simulink model "usv_model"  (R2015b)
settings: Solver=ode45  StartTime=0.0  StopTime=100000.0  RelTol=1e-3
model workspace (MAT data in the model file):
  B = 3.17
  Cb = 0.251
  Izz = 1
  L = 9.8
  d = 0.71
  m = 5540
undefined symbols (not defined in the file or in its folder): magnitude
libraries: simulink x2
settings Model: Creator=Administrator  LastModifiedBy=Administrator

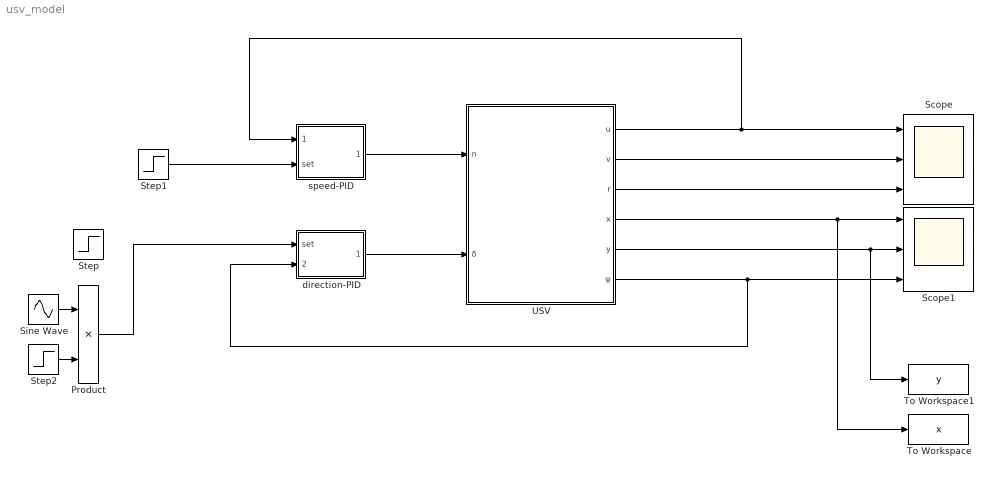
== system usv_model ==
  Product : Product
  Scope : Scope  NumInputPorts=3
  Scope1 : Scope  NumInputPorts=3
  Sine Wave : Sin  Amplitude=90  Frequency=1/5000  SampleTime=0
  Step : Step  Time=30000  After=50  SampleTime=0
  Step1 : Step  Time=0  After=0.1  SampleTime=0
  Step2 : Step  Time=60000  SampleTime=0
  To Workspace : ToWorkspace  VariableName=x  SampleTime=-1
  To Workspace1 : ToWorkspace  VariableName=y  SampleTime=-1
  USV : Subsystem
  direction-PID : Subsystem
  speed-PID : Subsystem
  wires:
  USV/5(y) -> To Workspace1/1, Scope1/2
  USV/4(x) -> To Workspace/1, Scope1/1
  USV/1(u) -> speed-PID/1(feedback), Scope/1
  USV/2(v) -> Scope/2
  USV/3(r) -> Scope/3
  USV/6(ψ) -> direction-PID/2(feedback), Scope1/3
  Sine Wave/1 -> Product/1
  Step2/1 -> Product/2
  Step1/1 -> speed-PID/2(set)
  speed-PID/1(output) -> USV/1(n)
  Product/1 -> direction-PID/1(set)
  direction-PID/1(output) -> USV/2(δ)

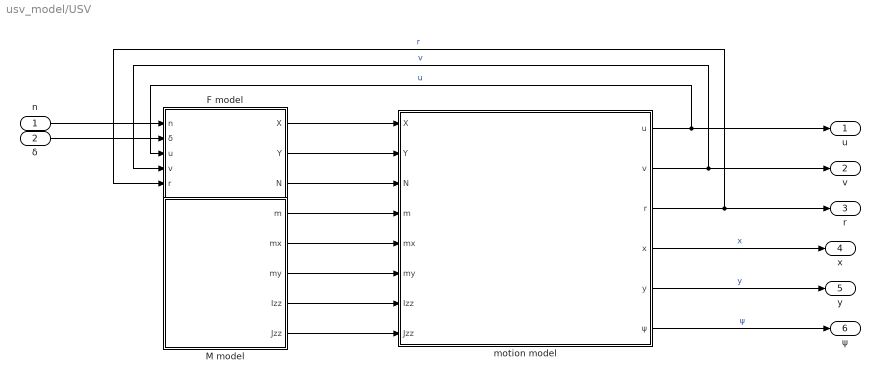
== system usv_model/USV ==
  n : Inport
  δ : Inport  Port=2
  F model : Subsystem
  M model : Subsystem
  motion model : Subsystem
  u : Outport
  v : Outport  Port=2
  r : Outport  Port=3
  x : Outport  Port=4
  y : Outport  Port=5
  ψ : Outport  Port=6
  wires:
  M model/5(Jzz) -> motion model/8(Jzz)
  M model/3(my) -> motion model/6(my)
  M model/1(m) -> motion model/4(m)
  F model/2(Y) -> motion model/2(Y)
  n/1 -> F model/1(n)
  δ/1 -> F model/2(δ)
  F model/1(X) -> motion model/1(X)
  motion model/1(u) -> u/1, F model/3(u)  "u"
  motion model/3(r) -> r/1, F model/5(r)  "r"
  motion model/2(v) -> v/1, F model/4(v)  "v"
  motion model/6(ψ) -> ψ/1  "ψ"
  F model/3(N) -> motion model/3(N)
  M model/2(mx) -> motion model/5(mx)
  M model/4(Izz) -> motion model/7(Izz)
  motion model/4(x) -> x/1  "x"
  motion model/5(y) -> y/1  "y"

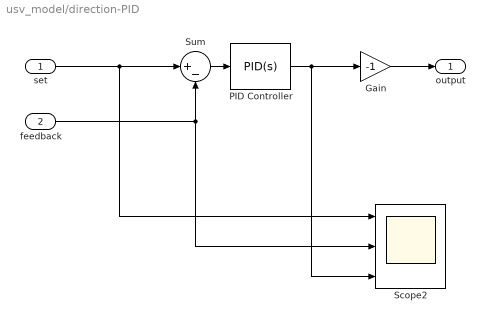
== system usv_model/direction-PID ==
  set : Inport
  feedback : Inport  Port=2
  Gain : Gain  Gain=-1
  PID Controller : simulink/Continuous/PID Controller  Controller=PID  TimeDomain=Continuous-time  SampleTime=-1  IntegratorMethod=Forward Euler  FilterMethod=Forward Euler  Form=Parallel  UseFilter=on  ControllerParametersSource=internal  P=1.2  I=0  D=0  N=5.45397025421619  InitialConditionSource=internal  InitialConditionForIntegrator=0  InitialConditionForFilter=0  ExternalReset=none  LimitOutput=on  UpperSaturationLimit=50  LowerSaturationLimit=-50  LinearizeAsGain=on  AntiWindupMode=none  Kb=1  TrackingMode=off  Kt=1  PParamMin=[]  PParamMax=[]  IParamMin=[]  IParamMax=[]  DParamMin=[]  DParamMax=[]  NParamMin=[]  NParamMax=[]  KbParamMin=[]  KbParamMax=[]  KtParamMin=[]  KtParamMax=[]  POutMin=[]  POutMax=[]  IOutMin=[]  IOutMax=[]  DOutMin=[]  DOutMax=[]  NOutMin=[]  NOutMax=[]  KbOutMin=[]  KbOutMax=[]  KtOutMin=[]  KtOutMax=[]  IntegratorOutMin=[]  IntegratorOutMax=[]  FilterOutMin=[]  FilterOutMax=[]  SumOutMin=[]  SumOutMax=[]  SumI1OutMin=[]  SumI1OutMax=[]  SumI2OutMin=[]  SumI2OutMax=[]  SumI3OutMin=[]  SumI3OutMax=[]  SumDOutMin=[]  SumDOutMax=[]  SaturationOutMin=[]  SaturationOutMax=[]  IntegratorContinuousStateAttributes=''  IntegratorStateMustResolveToSignalObject=off  IntegratorRTWStateStorageClass=Auto  FilterContinuousStateAttributes=''  FilterStateMustResolveToSignalObject=off  FilterRTWStateStorageClass=Auto  DifferentiatorICPrevScaledInput=0  DifferentiatorOutMin=[]  DifferentiatorOutMax=[]
  Scope2 : Scope  NumInputPorts=3
  Sum : Sum  Inputs=|+-
  output : Outport
  wires:
  PID Controller/1 -> Gain/1, Scope2/3
  Sum/1 -> PID Controller/1
  set/1 -> Scope2/1, Sum/1
  feedback/1 -> Scope2/2, Sum/2
  Gain/1 -> output/1

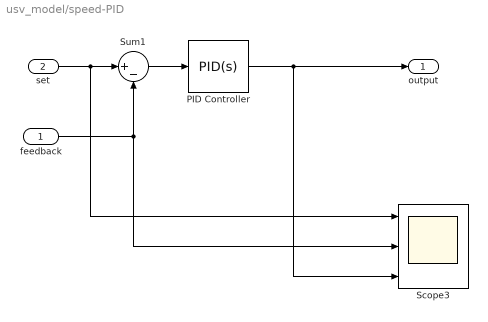
== system usv_model/speed-PID ==
  feedback : Inport
  set : Inport  Port=2
  PID Controller : simulink/Continuous/PID Controller  Controller=PID  TimeDomain=Continuous-time  SampleTime=-1  IntegratorMethod=Forward Euler  FilterMethod=Forward Euler  Form=Parallel  UseFilter=on  ControllerParametersSource=internal  P=3000  I=2  D=0  N=5.45397025421619  InitialConditionSource=internal  InitialConditionForIntegrator=0  InitialConditionForFilter=0  ExternalReset=none  LimitOutput=on  UpperSaturationLimit=2000  LowerSaturationLimit=0  LinearizeAsGain=on  AntiWindupMode=none  Kb=1  TrackingMode=off  Kt=1  PParamMin=[]  PParamMax=[]  IParamMin=[]  IParamMax=[]  DParamMin=[]  DParamMax=[]  NParamMin=[]  NParamMax=[]  KbParamMin=[]  KbParamMax=[]  KtParamMin=[]  KtParamMax=[]  POutMin=[]  POutMax=[]  IOutMin=[]  IOutMax=[]  DOutMin=[]  DOutMax=[]  NOutMin=[]  NOutMax=[]  KbOutMin=[]  KbOutMax=[]  KtOutMin=[]  KtOutMax=[]  IntegratorOutMin=[]  IntegratorOutMax=[]  FilterOutMin=[]  FilterOutMax=[]  SumOutMin=[]  SumOutMax=[]  SumI1OutMin=[]  SumI1OutMax=[]  SumI2OutMin=[]  SumI2OutMax=[]  SumI3OutMin=[]  SumI3OutMax=[]  SumDOutMin=[]  SumDOutMax=[]  SaturationOutMin=[]  SaturationOutMax=[]  IntegratorContinuousStateAttributes=''  IntegratorStateMustResolveToSignalObject=off  IntegratorRTWStateStorageClass=Auto  FilterContinuousStateAttributes=''  FilterStateMustResolveToSignalObject=off  FilterRTWStateStorageClass=Auto  DifferentiatorICPrevScaledInput=0  DifferentiatorOutMin=[]  DifferentiatorOutMax=[]
  Scope3 : Scope  NumInputPorts=3
  Sum1 : Sum  Inputs=|+-
  output : Outport
  wires:
  set/1 -> Sum1/1, Scope3/1
  PID Controller/1 -> output/1, Scope3/3
  Sum1/1 -> PID Controller/1
  feedback/1 -> Sum1/2, Scope3/2

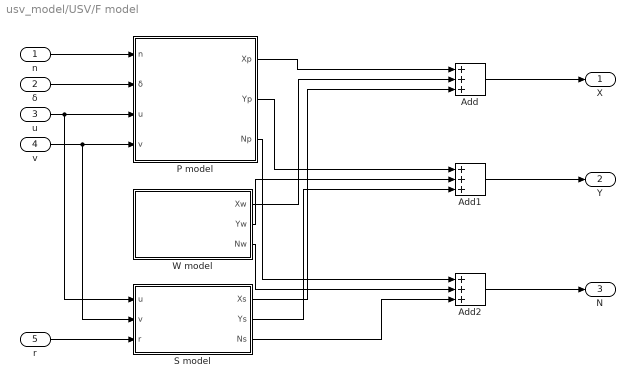
== system usv_model/USV/F model ==
  n : Inport
  δ : Inport  Port=2
  u : Inport  Port=3
  v : Inport  Port=4
  r : Inport  Port=5
  Add : Sum  Inputs=3
  Add1 : Sum  Inputs=3
  Add2 : Sum  Inputs=3
  P model : Subsystem
  S model : Subsystem
  W model : Subsystem
  X : Outport
  Y : Outport  Port=2
  N : Outport  Port=3
  wires:
  n/1 -> P model/1(n)
  δ/1 -> P model/2(δ)
  P model/1(Xp) -> Add/1
  W model/1(Xw) -> Add/2
  S model/1(Xs) -> Add/3
  P model/2(Yp) -> Add1/1
  W model/2(Yw) -> Add1/2
  S model/2(Ys) -> Add1/3
  P model/3(Np) -> Add2/1
  W model/3(Nw) -> Add2/2
  S model/3(Ns) -> Add2/3
  Add/1 -> X/1
  Add1/1 -> Y/1
  Add2/1 -> N/1
  u/1 -> S model/1(u), P model/3(u)
  v/1 -> S model/2(v), P model/4(v)
  r/1 -> S model/3(r)

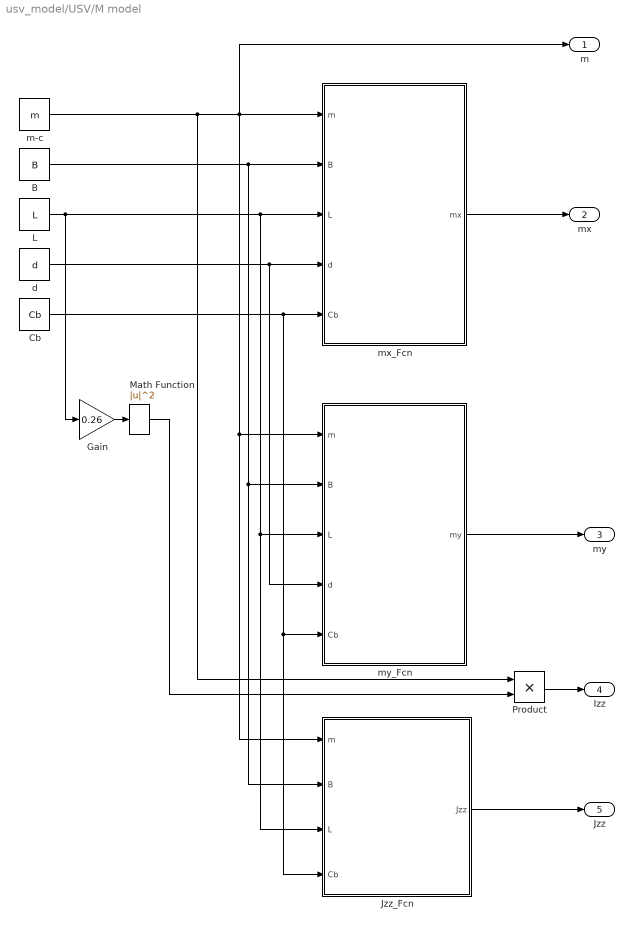
== system usv_model/USV/M model ==
  B : Constant  Value=B
  Cb : Constant  Value=Cb
  Gain : Gain  Gain=0.26
  Jzz_Fcn : MATLAB Function  TreatAsAtomicUnit=on
  L : Constant  Value=L
  Math Function : Math  Operator=magnitude^2  SaturateOnIntegerOverflow=on
  Product : Product
  d : Constant  Value=d
  m-c : Constant  Value=m
  mx_Fcn : MATLAB Function  TreatAsAtomicUnit=on
  my_Fcn : MATLAB Function  TreatAsAtomicUnit=on
  m : Outport
  mx : Outport  Port=2
  my : Outport  Port=3
  Izz : Outport  Port=4
  Jzz : Outport  Port=5
  wires:
  mx_Fcn/1(mx) -> mx/1
  d/1 -> my_Fcn/4(d), mx_Fcn/4(d)
  B/1 -> Jzz_Fcn/2(B), my_Fcn/2(B), mx_Fcn/2(B)
  my_Fcn/1(my) -> my/1
  Jzz_Fcn/1(Jzz) -> Jzz/1
  m-c/1 -> Product/1, m/1, Jzz_Fcn/1(m), my_Fcn/1(m), mx_Fcn/1(m)
  L/1 -> Gain/1, Jzz_Fcn/3(L), my_Fcn/3(L), mx_Fcn/3(L)
  Cb/1 -> Jzz_Fcn/4(Cb), my_Fcn/5(Cb), mx_Fcn/5(Cb)
  Gain/1 -> Math Function/1
  Product/1 -> Izz/1
  Math Function/1 -> Product/2

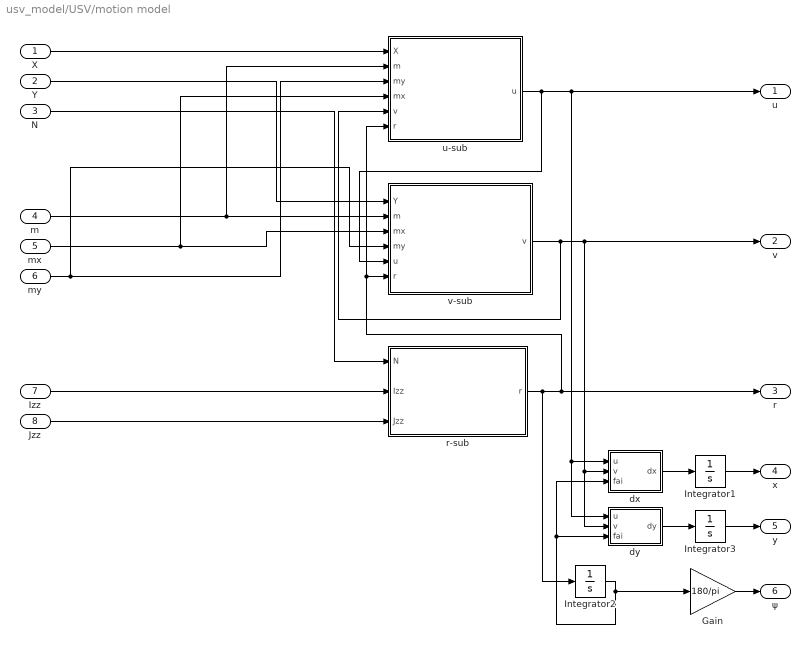
== system usv_model/USV/motion model ==
  X : Inport
  Y : Inport  Port=2
  N : Inport  Port=3
  m : Inport  Port=4
  mx : Inport  Port=5
  my : Inport  Port=6
  Izz : Inport  Port=7
  Jzz : Inport  Port=8
  Gain : Gain  Gain=180/pi
  Integrator1 : Integrator
  Integrator2 : Integrator
  Integrator3 : Integrator
  dx : MATLAB Function  TreatAsAtomicUnit=on
  dy : MATLAB Function  TreatAsAtomicUnit=on
  r-sub : Subsystem
  u-sub : Subsystem
  v-sub : Subsystem
  u : Outport
  v : Outport  Port=2
  r : Outport  Port=3
  x : Outport  Port=4
  y : Outport  Port=5
  ψ : Outport  Port=6
  wires:
  m/1 -> v-sub/2(m), u-sub/2(m)
  Y/1 -> v-sub/1(Y)
  r-sub/1(r) -> r/1, u-sub/6(r), v-sub/6(r), Integrator2/1
  Izz/1 -> r-sub/2(Izz)
  N/1 -> r-sub/1(N)
  Jzz/1 -> r-sub/3(Jzz)
  X/1 -> u-sub/1(X)
  my/1 -> u-sub/3(my), v-sub/4(my)
  mx/1 -> u-sub/4(mx), v-sub/3(mx)
  v-sub/1(v) -> dy/2(v), dx/2(v), v/1, u-sub/5(v)
  u-sub/1(u) -> u/1, dy/1(u), dx/1(u), v-sub/5(u)
  dy/1(dy) -> Integrator3/1
  dx/1(dx) -> Integrator1/1
  Integrator3/1 -> y/1
  Integrator1/1 -> x/1
  Gain/1 -> ψ/1
  Integrator2/1 -> Gain/1, dy/3(fai), dx/3(fai)

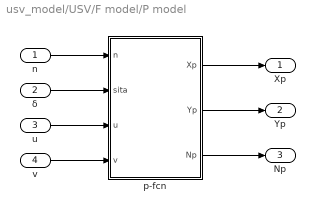
== system usv_model/USV/F model/P model ==
  n : Inport
  δ : Inport  Port=2
  u : Inport  Port=3
  v : Inport  Port=4
  p-fcn : MATLAB Function  TreatAsAtomicUnit=on
  Xp : Outport
  Yp : Outport  Port=2
  Np : Outport  Port=3
  wires:
  p-fcn/3(Np) -> Np/1
  p-fcn/2(Yp) -> Yp/1
  p-fcn/1(Xp) -> Xp/1
  n/1 -> p-fcn/1(n)
  δ/1 -> p-fcn/2(sita)
  u/1 -> p-fcn/3(u)
  v/1 -> p-fcn/4(v)

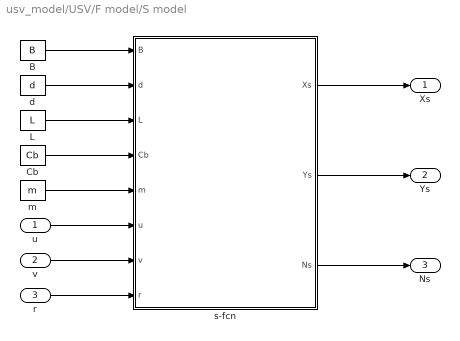
== system usv_model/USV/F model/S model ==
  u : Inport
  v : Inport  Port=2
  r : Inport  Port=3
  B : Constant  Value=B
  Cb : Constant  Value=Cb
  L : Constant  Value=L
  d : Constant  Value=d
  m : Constant  Value=m
  s-fcn : MATLAB Function  TreatAsAtomicUnit=on
  Xs : Outport
  Ys : Outport  Port=2
  Ns : Outport  Port=3
  wires:
  s-fcn/1(Xs) -> Xs/1
  s-fcn/2(Ys) -> Ys/1
  s-fcn/3(Ns) -> Ns/1
  B/1 -> s-fcn/1(B)
  d/1 -> s-fcn/2(d)
  L/1 -> s-fcn/3(L)
  u/1 -> s-fcn/6(u)
  v/1 -> s-fcn/7(v)
  r/1 -> s-fcn/8(r)
  Cb/1 -> s-fcn/4(Cb)
  m/1 -> s-fcn/5(m)

== system usv_model/USV/F model/W model ==
  n : Constant  Value=0
  n1 : Constant  Value=0
  n2 : Constant  Value=0
  Xw : Outport
  Yw : Outport  Port=2
  Nw : Outport  Port=3
  wires:
  n/1 -> Xw/1
  n2/1 -> Yw/1
  n1/1 -> Nw/1

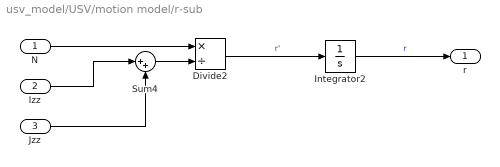
== system usv_model/USV/motion model/r-sub ==
  N : Inport
  Izz : Inport  Port=2
  Jzz : Inport  Port=3
  Divide2 : Product  Inputs=*/
  Integrator2 : Integrator
  Sum4 : Sum  Inputs=|++
  r : Outport
  wires:
  Sum4/1 -> Divide2/2
  Divide2/1 -> Integrator2/1  "r'"
  Integrator2/1 -> r/1  "r"
  N/1 -> Divide2/1
  Jzz/1 -> Sum4/2
  Izz/1 -> Sum4/1

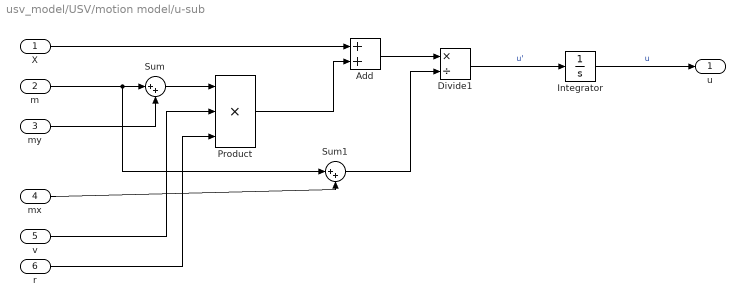
== system usv_model/USV/motion model/u-sub ==
  X : Inport
  m : Inport  Port=2
  my : Inport  Port=3
  mx : Inport  Port=4
  v : Inport  Port=5
  r : Inport  Port=6
  Add : Sum
  Divide1 : Product  Inputs=*/
  Integrator : Integrator
  Product : Product  Inputs=3
  Sum : Sum  Inputs=|++
  Sum1 : Sum  Inputs=|++
  u : Outport
  wires:
  Sum1/1 -> Divide1/2
  Divide1/1 -> Integrator/1  "u'"
  Integrator/1 -> u/1  "u"
  Sum/1 -> Product/1
  Add/1 -> Divide1/1
  my/1 -> Sum/2
  X/1 -> Add/1
  v/1 -> Product/2
  r/1 -> Product/3
  mx/1 -> Sum1/2
  m/1 -> Sum1/1, Sum/1
  Product/1 -> Add/2

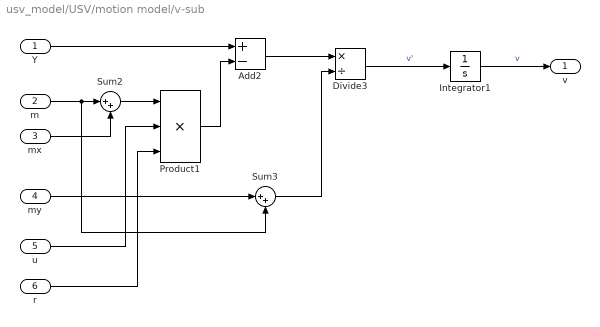
== system usv_model/USV/motion model/v-sub ==
  Y : Inport
  m : Inport  Port=2
  mx : Inport  Port=3
  my : Inport  Port=4
  u : Inport  Port=5
  r : Inport  Port=6
  Add2 : Sum  Inputs=+-
  Divide3 : Product  Inputs=*/
  Integrator1 : Integrator
  Product1 : Product  Inputs=3
  Sum2 : Sum  Inputs=|++
  Sum3 : Sum  Inputs=|++
  v : Outport
  wires:
  Sum3/1 -> Divide3/2
  my/1 -> Sum3/1
  r/1 -> Product1/3
  Product1/1 -> Add2/2
  m/1 -> Sum3/2, Sum2/1
  Sum2/1 -> Product1/1
  Y/1 -> Add2/1
  Add2/1 -> Divide3/1
  Divide3/1 -> Integrator1/1  "v'"
  Integrator1/1 -> v/1  "v"
  u/1 -> Product1/2
  mx/1 -> Sum2/2

== matlab function usv_model/USV/M model/my_Fcn ==
  data: m input; my output; B input; L input; d input; Cb input
function my = fcn(m, B, L, d, Cb)
%#codegen
temp = 0.882 - 0.54*Cb*(1-1.6*d/B) - 0.156*Cb*(1-0.673*Cb)*d/B + 0.826*d*L/(B*B)*(1-0.678*d/B) - 0.638*Cb*d*L/(B*B)*(1-0.619*d/B);
my = temp*m;

== matlab function usv_model/USV/M model/mx_Fcn ==
  data: m input; mx output; B input; L input; d input; Cb input
function mx = fcn(m, B, L, d, Cb)
%#codegen
temp = 0.398 + 11.97*Cb*(1+3.73*d/B) - 2.89*Cb*(1+1.13*d/B) + 0.175*Cb*(L/B)^2*(1+0.541*d/B) - 1.107*L*d/(B*B);
mx = temp*m/100;

== matlab function usv_model/USV/M model/Jzz_Fcn ==
  data: m input; Jzz output; B input; L input; Cb input
function Jzz = fcn(m, B, L, Cb)
%#codegen
temp = 33 - 76.85*Cb*(1-0.784*Cb) + 3.43*(1-0.63*Cb)*L/B;
Jzz = temp*m*L*L/100;

== matlab function usv_model/USV/motion model/dx ==
  data: u input; dx output; v input; fai input
function dx = fcn(u, v, fai)
%#codegen
dx = u*cos(fai) - v*sin(fai);

== matlab function usv_model/USV/motion model/dy ==
  data: u input; dy output; v input; fai input
function dy = fcn(u, v, fai)
%#codegen
dy = u*sin(fai) + v*cos(fai);

== matlab function usv_model/USV/F model/P model/p-fcn ==
  data: n input; Xp output; sita input; Yp output; Np output; u input; v input
function [Xp, Yp, Np]= fcn(n, sita, u, v)
%#codegen
Q = 1000;  %水密度
A = 0.95;         %动量影响因子
beita = A*A;      %进口动能利用系数
C = 10;            %功率特性系数，单位千瓦
g = 9.8;          %重力加速度
np = 0.8;         %推进泵效率
Aj = pi*(0.25/2)^2;    %喷口处面积
Ain = 1.6*0.52;   %入口处管道面积
Aw = pi*0.5^2;    %弯道处管道面积
Ein = 0.01;       %进口损失系数
En = 0.02;        %水力损失系数
E0 = 0.01;        %弯道损失系数
h = 0.6;          %喷口高度损失

Xt = 3;    %推力作用点在舰体坐标系下的坐标

sita = sita*pi/180;
Vs = (u^2+v^2)^(1/2); %船的航速

p = Q*Aj*(1/2+Ein/2*(Aj/Ain)^2+En/2+E0/2*(Aj/Aw)^2);
q = Q*g*Aj*(h-beita*Vs^2/(2*g));
r = -C*(n/1000)^3*np;

%p = g*(h-beita*Vs^2/(2*g))/(1/2+Ein/2*(Aj/Ain)^2+En/2+E0/2*(Aj/Aw)^2);
%q = -C*(n/1000)^3*np/(Q*Aj*(1/2+Ein/2*(Aj/Ain)^2+En/2+E0/2*(Aj/Aw)^2));
%Vj = (-q/2-((q/2)^2+(p/3)^3)^(1/2))^(1/3) + (-q/2+((q/2)^2+(p/3)^3)^(1/2))^(1/3);
V = roots([p 0 q r]);
Vj = 0;

for i=1:size(V,1)
    if imag(V(i)) < 10^(-10)
        Vj = real(V(i));
    end
end
Xp = Q*Aj*Vj*(Vj-A*Vs)*cos(sita);
Yp = Q*Aj*Vj*(Vj-A*Vs)*sin(sita);
Np = Yp*Xt;

== matlab function usv_model/USV/F model/S model/s-fcn ==
  data: B input; Xs output; d input; L input; Cb input; m input; Ys output; Ns output; u input; v input; r input
function [Xs, Ys, Ns]= fcn(B, d, L, Cb, m, u, v, r)
%#codegen
P = 1000;
K = 2*d/L;
dA = 0.67;
df = 0.72;
d1 = dA-df;
d2 = (dA+df)/2;
t = d1/d2; 
U = (u^2+v^2)^(1/2);
deta = m/1025;
S = (3.14^(deta/3)+0.5*L)^(1/3);
vv = 1.07854*10^(-6);
Re = L*U/vv;
Cf = 0.075/(log10(Re)-2)^2;
Ks = 150*10^(-6);
deCf = (105*(Ks/L)^(1/3)-0.64)*10^(-3);

Xu = -0.5*P*S*u^2*(Cf+deCf);
Yv = -1/2*P*L*d*U*((0.5*pi*K+1.4*Cb*B/L)*(1+0.67*t/d));
Yr = 1/2*P*L*L*d*U*(0.25*pi*K*(1+0.8*t/d));
Nv = -1/2*P*L*L*d*U*(K-0.27*(0.5*pi+1.4*Cb*B/L)*t/d);
Nr = 1/2*P*L^3*d*U*(-(0.54*K-K^2)*(1+0.3*t/d));

Xs = Xu;
Ys = Yv*v + Yr*r;
Ns = Nv*v + Nr*r;
